simulink model "NoiseComparison"  (R2023b)
settings: Solver=FixedStepDiscrete  StartTime=0.0  StopTime=1000  FixedStep=Tp  MaxStep=0.01  RelTol=1e-3  EnableMultiTasking=on
values from neighbouring files (symbols this model uses):
  Tp = 0.001    [Zad1_3.m]    (also in Zad_2_1.m; zad21.m)
libraries: simulink x1
settings Model: Creator=MMM-PP  LastModifiedBy=falat
settings SolverCC: AlgebraicLoopSolver=TrustRegion
settings DataIOCC: LimitDataPoints=on  SaveFormat=Array  SignalLoggingSaveFormat=ModelDataLogs  ReturnWorkspaceOutputs=off
settings OptimizationCC: InitFltsAndDblsToZero=on  LifeSpan=inf
settings DebuggingCC: SaveWithParameterizedLinksMsg=none  UnderspecifiedInitializationDetection=Classic  MergeDetectMultiDrivingBlocksExec=none  SignalResolutionControl=TryResolveAllWithWarning  SolverPrmCheckMsg=warning  MultiTaskDSMMsg=warning  MultiTaskCondExecSysMsg=none  FcnCallInpInsideContextMsg=warning  UnconnectedInputMsg=warning  UnconnectedOutputMsg=warning  UnconnectedLineMsg=warning  SFUnexpectedBacktrackingDiag=warning  SFNoUnconditionalDefaultTransitionDiag=warning  ArithmeticOperatorsInVariantConditions=warning
settings HardwareCC: ProdBitPerPointer=32  ProdBitPerSizeT=32  ProdBitPerPtrDiffT=32  ProdLargestAtomicFloat=None  ProdIntDivRoundTo=Undefined  ProdEndianess=Unspecified  ProdWordSize=32  ProdHWDeviceType=32-bit Generic
settings ModelReferenceCC: EnableRefExpFcnMdlSchedulingChecks=on  PropagateSignalLabelsOutOfModel=off
settings SFSimCC: SimUseLocalCustomCode=off  CustomCodeUndefinedFunction=UseInterfaceOnly
settings RTWCC: RTWUseLocalCustomCode=off
settings CodeAppCC: StateflowObjectComments=on
settings GRTTargetCC: TargetFcnLib=ansi_tfl_tmw.mat  TargetLangStandard=C89/C90 (ANSI)  CombineOutputUpdateFcns=off  GRTInterface=on
settings ConfigComp: CovMetricSettings=dw  CovSaveCumulativeToWorkspaceVar=on  CovSaveSingleToWorkspaceVar=on  CovExternalEMLEnable=off

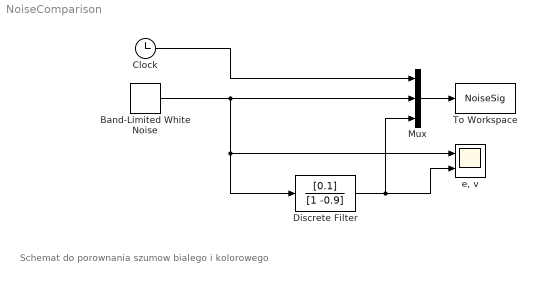
== system NoiseComparison ==
  note: Schemat do porownania szumow bialego i kolorowego
  Band-Limited White Noise : simulink/Sources/Band-Limited White Noise  Cov=[0.5]*Tp  Ts=Tp  seed=[23341]
  Clock : Clock
  Discrete Filter : DiscreteFilter  Numerator=[0.1]  Denominator=[1 -0.9]  SampleTime=Tp
  Mux : Mux  Inputs=3
  To Workspace : ToWorkspace  VariableName=NoiseSig  SampleTime=-1
  "e, v" : Scope  NumInputPorts=2
  wires:
  Mux/1 -> To Workspace/1
  Clock/1 -> Mux/1
  Band-Limited White Noise/1 -> Mux/2, "e, v"/1, Discrete Filter/1
  Discrete Filter/1 -> "e, v"/2, Mux/3
